simulink model "PID_simulink"  (Simulink 7.8)
settings: Solver=ode23s  StartTime=0.0  StopTime=10  RelTol=1e-10  AbsTol=1e-10
values from neighbouring files (symbols this model uses):
  epsilon = 0.00001    (= 1e-05)    [Pid_variabili_grafici.m]
  Kd = Kp*Td    (= 0.02712)    [Pid_variabili_grafici.m]
  Ki = Kp*0.1*140    (= 18.984)    [Pid_variabili_grafici.m]
  Kp = 0.6*Kp_signed    (= 1.356)    [Pid_variabili_grafici.m]
  omega_n1 = 2 * pi/0.042    (= 149.599650171)    [Pid_variabili_grafici.m]
  omega_n2 = 2 * pi/0.05    (= 125.663706144)    [Pid_variabili_grafici.m]
  zita1 = 0.46    [Pid_variabili_grafici.m]
  zita2 = 0.8    [Pid_variabili_grafici.m]
settings Model: Creator=danielecarnevale  LastModifiedBy=dAnIeLe

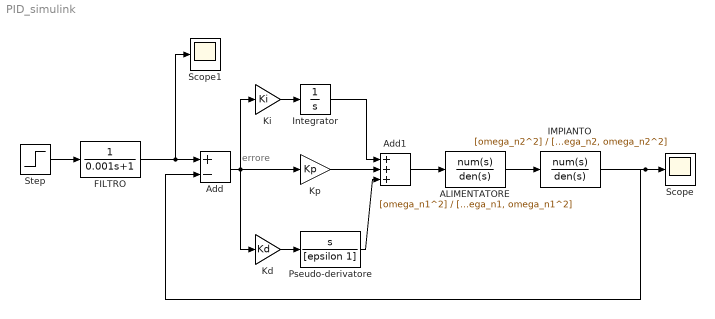
== system PID_simulink ==
  note: errore
  ALIMENTATORE : TransferFcn  Numerator=[omega_n1^2]  Denominator=[1, 2*zita1*omega_n1, omega_n1^2]  ContinuousStateAttributes='ALIMENTATORE'
  Add : Sum  Inputs=+-
  Add1 : Sum  Inputs=+++
  FILTRO : TransferFcn  Denominator=[0.001 1]  ContinuousStateAttributes='ALIMENTATORE'
  IMPIANTO : TransferFcn  Numerator=[omega_n2^2]  Denominator=[1, 2*zita2*omega_n2, omega_n2^2]  ContinuousStateAttributes='SPIRE'
  Integrator : Integrator
  Kd : Gain  Gain=Kd
  Ki : Gain  Gain=Ki
  Kp : Gain  Gain=Kp
  Pseudo-derivatore : TransferFcn  Numerator=[1 0]  Denominator=[epsilon 1]  ContinuousStateAttributes='ALIMENTATORE'
  Scope : Scope
      settings: YMin=0.1  YMax=1.4
  Scope1 : Scope
  Step : Step  SampleTime=0
  wires:
  ALIMENTATORE/1 -> IMPIANTO/1
  Add/1 -> Kp/1, Kd/1, Ki/1
  IMPIANTO/1 -> Add/2, Scope/1
  Step/1 -> FILTRO/1
  Kp/1 -> Add1/2
  Integrator/1 -> Add1/1
  Pseudo-derivatore/1 -> Add1/3
  Add1/1 -> ALIMENTATORE/1
  Kd/1 -> Pseudo-derivatore/1
  Ki/1 -> Integrator/1
  FILTRO/1 -> Add/1, Scope1/1
